simulink model "pendule_inv_capteur_etu"  (R2017a)
settings: Solver=VariableStepAuto  StartTime=t0  StopTime=tf  RelTol=1e-3
undefined symbols (not defined in the file): g, K, l, ue, x0, xe
settings Model: Creator=cmaurice  LastModifiedBy=cmaurice

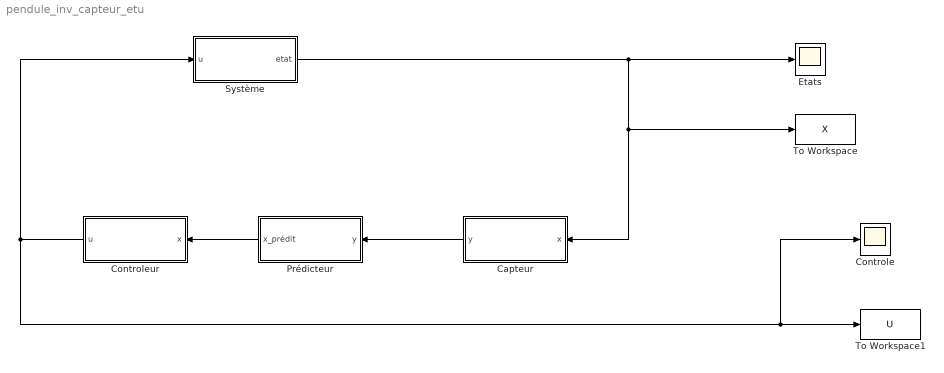
== system pendule_inv_capteur_etu ==
  Capteur : Subsystem
  Controle : Scope
  Controleur : Subsystem
  Etats : Scope
  Prédicteur : Subsystem
  Système : Subsystem
  To Workspace : ToWorkspace  VariableName=X  SaveFormat=Timeseries  SampleTime=-1
  To Workspace1 : ToWorkspace  VariableName=U  SaveFormat=Timeseries  SampleTime=-1
  wires:
  Prédicteur/1(x_prédit) -> Controleur/1(x)
  Capteur/1(y) -> Prédicteur/1(y)
  Système/1(etat) -> Etats/1, To Workspace/1, Capteur/1(x)
  Controleur/1(u) -> Controle/1, To Workspace1/1, Système/1(u)

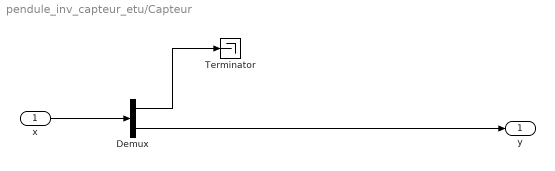
== system pendule_inv_capteur_etu/Capteur ==
  x : Inport
  Demux : Demux  Outputs=2
  Terminator : Terminator
  y : Outport
  wires:
  Demux/1 -> Terminator/1
  Demux/2 -> y/1
  x/1 -> Demux/1

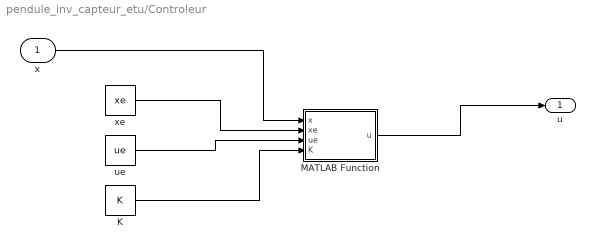
== system pendule_inv_capteur_etu/Controleur ==
  x : Inport
  K : Constant  Value=K
  MATLAB Function : MATLAB Function  TreatAsAtomicUnit=on
  ue : Constant  Value=ue
  xe : Constant  Value=xe
  u : Outport
  wires:
  x/1 -> MATLAB Function/1(x)
  ue/1 -> MATLAB Function/3(ue)
  K/1 -> MATLAB Function/4(K)
  xe/1 -> MATLAB Function/2(xe)
  MATLAB Function/1(u) -> u/1

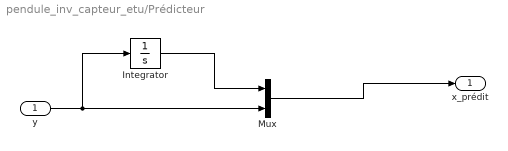
== system pendule_inv_capteur_etu/Prédicteur ==
  y : Inport
  Integrator : Integrator  InitialCondition=x0(1)
  Mux : Mux  Inputs=2
  x_prédit : Outport
  wires:
  y/1 -> Integrator/1, Mux/2
  Integrator/1 -> Mux/1
  Mux/1 -> x_prédit/1

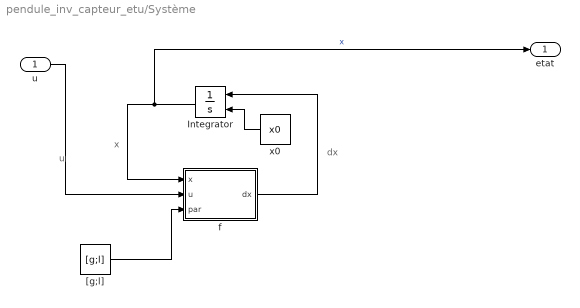
== system pendule_inv_capteur_etu/Système ==
  note: dx
  note: x
  note: u
  u : Inport
  Integrator : Integrator  InitialConditionSource=external
  "[g;l] " : Constant  Value=[g;l]
  f : MATLAB Function  TreatAsAtomicUnit=on
  "x0 " : Constant  Value=x0
  etat : Outport
  wires:
  "x0 "/1 -> Integrator/2
  Integrator/1 -> etat/1, f/1(x)  "x"
  f/1(dx) -> Integrator/1
  "[g;l] "/1 -> f/3(par)
  u/1 -> f/2(u)

== matlab function pendule_inv_capteur_etu/Système/f ==
  data: x input; u input; dx output; par input
function dx = fcn(x,u,par)
g = par(1);
l = par(2);
dx = [x(2); (g/l)*sin(x(1))-(cos(x(1))*u)/l];

== matlab function pendule_inv_capteur_etu/Controleur/MATLAB Function ==
  data: x input; u output; xe input; ue input; K input
function u = fcn(x,xe,ue,K)
u = ue + K(:)'*(x(:)-xe(:));
